simulink model "mpc"  (R2021a)
settings: Solver=VariableStepAuto  StartTime=0.0  StopTime=2500  RelTol=1e-3
libraries: mpclib x1
settings Model: Creator=jessilbijou  LastModifiedBy=jessilbijou

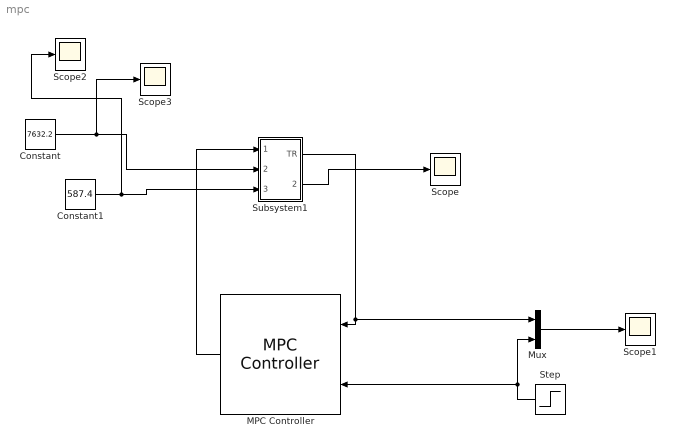
== system mpc ==
  Constant : Constant  Value=7632.2
  Constant1 : Constant  Value=587.4
  MPC Controller : mpclib/MPC Controller  SCDEnableBlockLinearizationSpecification=on  mpcobj=mpc1  is_multiple=0  enable_value=0  return_u0=off  updateMPCinCallerWorkspace=on  md_inport=off  mv_inport=off  uref_inport=off  return_cost=off  return_mvseq=off  return_qpstatus=off  return_xseq=off  return_state=off  return_ovseq=off  state_inport=off  umin_inport=off  umax_inport=off  ymin_inport=off  ymax_inport=off  cc_inport=off  ywt_inport=off  uwt_inport=off  duwt_inport=off  rhoeps_inport=off  pm_inport=off  MaximumP=10  HorizonChoice=FixedHorizon  n_ts=1  n_p=20  n_mv=1  n_md=0  n_ud=0  n_mo=1  n_uo=0  BlockDataType=double  SampleTimeInherited=off  switch_inport=off
  Mux : Mux  Inputs=2
  Scope{,1..3} (4 alike) : Scope
  Step : Step  Time=800  Before=415  After=418  SampleTime=0
  Subsystem1 : Subsystem
  wires:
  Mux/1 -> Scope1/1
  Step/1 -> MPC Controller/2, Mux/2
  Subsystem1/2(Out1) -> Scope/1
  Subsystem1/1(TR) -> MPC Controller/1, Mux/1
  MPC Controller/1 -> Subsystem1/1(In1)
  Constant/1 -> Scope3/1, Subsystem1/2(In2)
  Constant1/1 -> Scope2/1, Subsystem1/3(In3)

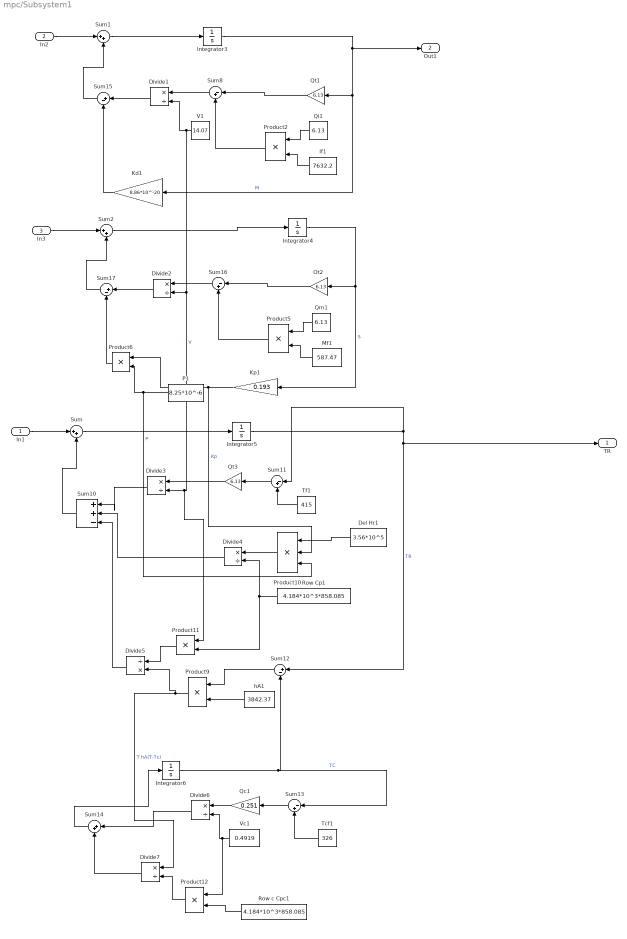
== system mpc/Subsystem1 ==
  In1 : Inport
  In2 : Inport  Port=2
  In3 : Inport  Port=3
  Del Hr1 : Constant  Value=3.56*10^5
  Divide{1..4,6..7} (6 alike) : Product  Inputs=*/
  Divide5 : Product  Inputs=/*
  If1 : Constant  Value=7632.2
  Integrator3 : Integrator  InitialCondition=7632.2
  Integrator4 : Integrator  InitialCondition=587.47
  Integrator5 : Integrator  InitialCondition=415
  Integrator6 : Integrator  InitialCondition=326
  Kd1 : Gain  Gain=8.86*10^-20
  Kp1 : Gain  Gain=0.193
  Mf1 : Constant  Value=587.47
  Ot2 : Gain  Gain=6.13
  P1 : Constant  Value=8.25*10^-6
  Product10 : Product  Inputs=3
  Product{2,5..6,9,11..12} (6 alike) : Product
  Qc1 : Gain  Gain=0.251
  Qi1 : Constant  Value=6.13
  Qm1 : Constant  Value=6.13
  Qt1 : Gain  Gain=6.13
  Qt3 : Gain  Gain=6.13
  Row Cp1 : Constant  Value=4.184*10^3*858.085
  Row c Cpc1 : Constant  Value=4.184*10^3*858.085
  Sum{,1..2,14} (4 alike) : Sum  Inputs=|++
  Sum10 : Sum  Inputs=|++-
  Sum{8,11,13,16} (4 alike) : Sum  Inputs=|-+
  Sum12 : Sum  Inputs=|+-
  Sum15 : Sum  Inputs=|+-
  Sum17 : Sum  Inputs=|+-
  Tcf1 : Constant  Value=326
  Tf1 : Constant  Value=415
  V1 : Constant  Value=14.07
  Vc1 : Constant  Value=0.4919
  hA1 : Constant  Value=3842.37
  TR : Outport
  Out1 : Outport  Port=2
  wires:
  Qm1/1 -> Product5/1
  Sum12/1 -> Product9/1
  Integrator5/1 -> TR/1, Sum12/1, Sum11/1  "TR"
  Ot2/1 -> Sum16/1
  Product11/1 -> Divide5/1
  Divide4/1 -> Sum10/2
  Sum16/1 -> Divide2/1
  Del Hr1/1 -> Product10/1
  Qi1/1 -> Product2/1
  Divide5/1 -> Sum10/3
  hA1/1 -> Product9/2
  Row c Cpc1/1 -> Product12/2
  Product10/1 -> Divide4/1
  Kd1/1 -> Sum15/2
  If1/1 -> Product2/2
  Divide3/1 -> Sum10/1
  Product6/1 -> Sum17/2
  Mf1/1 -> Product5/2
  Qt1/1 -> Sum8/1
  Kp1/1 -> Product6/1, Product10/2  "Kp"
  Tcf1/1 -> Sum13/2
  Integrator3/1 -> Out1/1, Kd1/1, Qt1/1  "M"
  Product9/1 -> Divide5/2, Divide7/1  "T hA(T-Tc)"
  Row Cp1/1 -> Product11/2, Divide4/2
  Sum11/1 -> Qt3/1
  Divide1/1 -> Sum15/1
  Product5/1 -> Sum16/2
  P1/1 -> Product6/2, Product10/3  "P"
  Vc1/1 -> Product12/1, Divide6/2
  Product2/1 -> Sum8/2
  V1/1 -> Product11/1, Divide3/2, Divide2/2, Divide1/2  "V"
  Sum8/1 -> Divide1/1
  Integrator4/1 -> Kp1/1, Ot2/1  "S"
  Divide6/1 -> Sum14/1
  Divide2/1 -> Sum17/1
  Divide7/1 -> Sum14/2
  Tf1/1 -> Sum11/2
  Qc1/1 -> Divide6/1
  Sum13/1 -> Qc1/1
  Product12/1 -> Divide7/2
  Integrator6/1 -> Sum13/1, Sum12/2  "TC"
  Qt3/1 -> Divide3/1
  Sum14/1 -> Integrator6/1
  Sum/1 -> Integrator5/1
  In1/1 -> Sum/1
  Sum10/1 -> Sum/2
  Sum1/1 -> Integrator3/1
  Sum15/1 -> Sum1/2
  In2/1 -> Sum1/1
  Sum2/1 -> Integrator4/1
  In3/1 -> Sum2/1
  Sum17/1 -> Sum2/2
